simulink library "SimplusGT"  (R2022b)
settings: Solver=ode45  StartTime=0.0  StopTime=10.0  RelTol=1e-3
values from neighbouring files (symbols this model uses):
  ang_r = u(3)    [Class_GridFollowingVSI.m]    (also in Class_GridFollowingVSI_Disturb.m; Class_GridFollowingVSI_old.m)
  Cf = obj.Para(3)    [Class_GridFormingVSI.m]
  Lc = obj.Para(4)    [Class_GridFormingVSI.m]
  Lf = obj.Para(1)    [Class_GridFormingVSI.m]
  P_dc = u(4)    [Class_GridFollowingVSI.m]    (also in Class_GridFollowingVSI_Disturb.m; Class_GridFollowingVSI_old.m)
  Ts = []    [Class_Model_Advance.m]
  V = obj.PowerFlow(3)    [Class_GridFollowingVSI.m]    (also in Class_GridFollowingVSI_Disturb.m; Class_GridFollowingVSI_old.m; Class_GridFormingVSI.m; Class_InfiniteBus.m)
  x0 = []    [Class_Model_Advance.m]
undefined symbols (not defined in the file or in its folder): DiscIntNeverNeededParam, initial, m, OtherInputs, Sbase, t0, Tm_pu, Vbase, w_droop, w_i, w_pll, w_tau, w_v, Wbase, wc, wfil, Ybase, Zbase
libraries: spsVoltageMeasurementLib x107, spsCurrentMeasurementLib x92, spsControlledCurrentSourceLib x57, spsThreePhaseSeriesRLCBranchLib x29, spsControlledVoltageSourceLib x19, spsSeriesRLCBranchLib x15, SimplexPS_2015a x6, spsThreePhaseParallelRLCBranchLib x3, spsThreePhaseBreakerLib x2, $bdroot x1
(part 4 of 8)

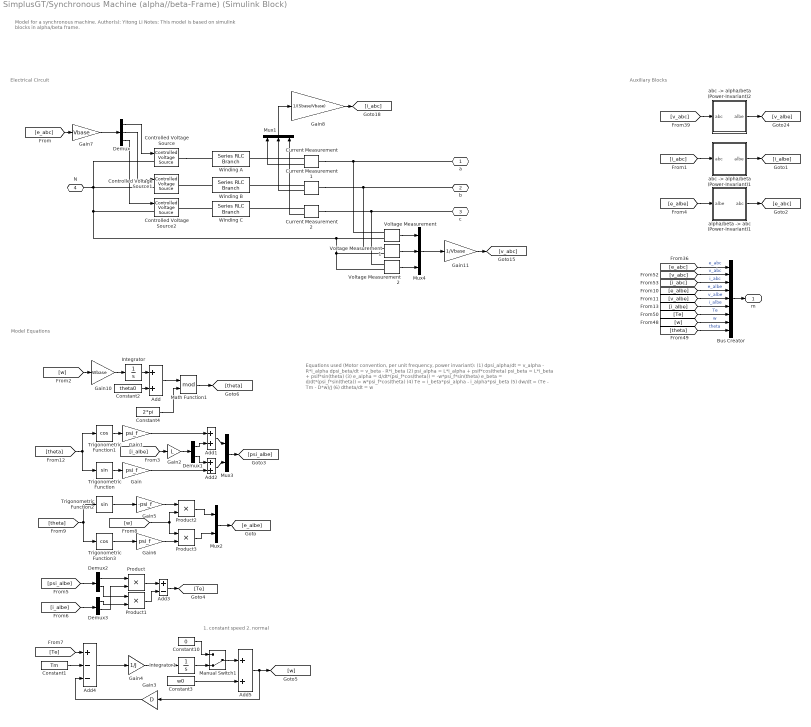
== system SimplusGT/Synchronous Machine (alpha//beta-Frame) (Simulink Block) ==
  note: 1. constant speed
      | 2. normal
  note: Auxiliary Blocks
  note: Model Equations
  note: Electrical Circuit
  note: Equations used
      | (Motor convention, per unit frequency, power invariant):
      |
      | (1) dpsi_alpha/dt = v_alpha - R*i_alpha
      | dpsi_beta/dt = v_beta - R*i_beta
      |
      | (2) psi_alpha = L*i_alpha + psif*cos(theta)
      | psi_beta = L*i_beta + psif*sin(theta)
      |
      | (3) e_alpha = d/dt*(psi_f*cos(theta)) = -w*psi_f*sin(theta)
      | e_beta = d/dt*(psi_f*sin(theta)) = w*psi_f*cos(theta)
      |
      | (4) Te = i_beta*psi_alpha - i_alpha*psi_beta
      | (5) dw/dt = (Te - Tm - D*w)/J
      | (6) dtheta/dt = w
  note: Model for a synchronous machine.
      |
      | Author(s): Yitong Li
      |
      | Notes:
      |
      | This model is based on simulink blocks in alpha/beta frame.
  Add{,1..2,5} (4 alike) : Sum
  Add3 : Sum  Inputs=+-
  Add4 : Sum  Inputs=+--
  Bus Creator : BusCreator  Inputs=9
  Constant1 : Constant  Value=Tm
  Constant10 : Constant  Value=0
  Constant2 : Constant  Value=theta0
  Constant3 : Constant  Value=w0
  Constant4 : Constant  Value=2*pi
  Controlled Voltage Source : spsControlledVoltageSourceLib/Controlled Voltage Source  Initialize=on  Source_Type=AC  Amplitude=0  Phase=0  Frequency=0  Measurements=None
  Controlled Voltage Source1 : spsControlledVoltageSourceLib/Controlled Voltage Source  Initialize=on  Source_Type=AC  Amplitude=0  Phase=0  Frequency=0  Measurements=None
  Controlled Voltage Source2 : spsControlledVoltageSourceLib/Controlled Voltage Source  Initialize=on  Source_Type=AC  Amplitude=0  Phase=0  Frequency=0  Measurements=None
  Current Measurement : spsCurrentMeasurementLib/Current Measurement  PhasorSimulation=off  OutputType=Complex  PSBequivalent=0
  Current Measurement1 : spsCurrentMeasurementLib/Current Measurement  PhasorSimulation=off  OutputType=Complex  PSBequivalent=0
  Current Measurement2 : spsCurrentMeasurementLib/Current Measurement  PhasorSimulation=off  OutputType=Complex  PSBequivalent=0
  Demux : Demux  Outputs=3
  Demux1 : Demux  Outputs=2
  Demux2 : Demux  Outputs=2
  Demux3 : Demux  Outputs=2
  Gain : Gain  Gain=psi_f
  Gain1 : Gain  Gain=psi_f
  Gain10 : Gain  Gain=Wbase
  Gain11 : Gain  Gain=1/Vbase
  Gain2 : Gain  Gain=L
  Gain3 : Gain  Gain=D
  Gain4 : Gain  Gain=1/J
  Gain5 : Gain  Gain=-psi_f
  Gain6 : Gain  Gain=psi_f
  Gain7 : Gain  Gain=Vbase
  Gain8 : Gain  Gain=1/(Sbase/Vbase)
  Integrator : Integrator
  Integrator1 : Integrator
  Manual Switch1 : ManualSwitch  CurrentSetting=0
  Math Function1 : Math  Operator=mod  SignedPower=on
  Mux1 : Mux  Inputs=3
  Mux2 : Mux  Inputs=2
  Mux3 : Mux  Inputs=2
  Mux4 : Mux  Inputs=3
  Product{,1..3} (4 alike) : Product
  Trigonometric Function : Trigonometry
  Trigonometric Function1 : Trigonometry  Operator=cos
  Trigonometric Function2 : Trigonometry
  Trigonometric Function3 : Trigonometry  Operator=cos
  Voltage Measurement : spsVoltageMeasurementLib/Voltage Measurement  PhasorSimulation=off  OutputType=Complex  PSBequivalent=0
  Voltage Measurement1 : spsVoltageMeasurementLib/Voltage Measurement  PhasorSimulation=off  OutputType=Complex  PSBequivalent=0
  Voltage Measurement2 : spsVoltageMeasurementLib/Voltage Measurement  PhasorSimulation=off  OutputType=Complex  PSBequivalent=0
  Winding A : spsSeriesRLCBranchLib/Series RLC Branch  LConnTagsString=__new0  RConnTagsString=__new0  BranchType=RL  Resistance=R*(Vbase^2)/Sbase  Inductance=L*(Vbase^2)/Sbase/Wbase  SetiL0=off  InitialCurrent=ia0  Capacitance=1e-6  Setx0=off  InitialVoltage=0  Measurements=None
  Winding B : spsSeriesRLCBranchLib/Series RLC Branch  LConnTagsString=__new0  RConnTagsString=__new0  BranchType=RL  Resistance=R*(Vbase^2)/Sbase  Inductance=L*(Vbase^2)/Sbase/Wbase  SetiL0=off  InitialCurrent=ia0  Capacitance=1e-6  Setx0=off  InitialVoltage=0  Measurements=None
  Winding C : spsSeriesRLCBranchLib/Series RLC Branch  LConnTagsString=__new0  RConnTagsString=__new0  BranchType=RL  Resistance=R*(Vbase^2)/Sbase  Inductance=L*(Vbase^2)/Sbase/Wbase  SetiL0=off  InitialCurrent=ia0  Capacitance=1e-6  Setx0=off  InitialVoltage=0  Measurements=None
  "abc -> alpha/beta (Power-Invariant)1" : Subsystem  AncestorBlock=|
      | SimplusGT/abc -> alpha//beta
      | (Power-Invariant)
      settings: LibrarySourceBlock=|
      | SimplusGT/abc -> alpha//beta
      | (Power-Invariant)
  "abc -> alpha/beta (Power-Invariant)2" : Subsystem  AncestorBlock=|
      | SimplusGT/abc -> alpha//beta
      | (Power-Invariant)
      settings: LibrarySourceBlock=|
      | SimplusGT/abc -> alpha//beta
      | (Power-Invariant)
  "alpha/beta -> abc (Power-Invariant)1" : Subsystem  AncestorBlock=|
      | SimplusGT/alpha//beta -> abc
      | (Power-Invariant)
      settings: LibrarySourceBlock=|
      | SimplusGT/alpha//beta -> abc
      | (Power-Invariant)
  a : PMIOPort  Side=Left
  b : PMIOPort  Port=2  Side=Left
  c : PMIOPort  Port=3  Side=Left
  N : PMIOPort  Port=4  Side=Left
  m : Outport
  wires:
  Current Measurement/1 -> Mux1/1
  Current Measurement1/1 -> Mux1/2
  Current Measurement2/1 -> Mux1/3
  Mux1/1 -> Gain8/1
  [e_abc] -> Gain7/1
  Demux/1 -> Controlled Voltage Source/1
  Demux/2 -> Controlled Voltage Source1/1
  Demux/3 -> Controlled Voltage Source2/1
  [i_abc] -> "abc -> alpha/beta (Power-Invariant)1"/1(abc)
  "abc -> alpha/beta (Power-Invariant)1"/1(albe) -> [i_albe]
  [w] -> Gain10/1
  Integrator/1 -> Add/1
  Constant2/1 -> Add/2
  Trigonometric Function1/1 -> Gain1/1
  Trigonometric Function/1 -> Gain/1
  [i_albe] -> Gain2/1
  Demux1/1 -> Add1/2
  Demux1/2 -> Add2/1
  Gain2/1 -> Demux1/1
  Gain1/1 -> Add1/1
  Gain/1 -> Add2/2
  Product2/1 -> Mux2/1
  Product3/1 -> Mux2/2
  Mux2/1 -> [e_albe]
  [e_albe] -> "alpha/beta -> abc (Power-Invariant)1"/1(albe)
  "alpha/beta -> abc (Power-Invariant)1"/1(abc) -> [e_abc]
  Add1/1 -> Mux3/1
  Add2/1 -> Mux3/2
  Mux3/1 -> [psi_albe]
  [psi_albe] -> Demux2/1
  [i_albe] -> Demux3/1
  Demux2/1 -> Product/1
  Demux3/2 -> Product/2
  Demux3/1 -> Product1/2
  Demux2/2 -> Product1/1
  Product/1 -> Add3/1
  Product1/1 -> Add3/2
  Add3/1 -> [Te]
  [Te] -> Add4/1
  Constant1/1 -> Add4/2
  Add4/1 -> Gain4/1
  Gain3/1 -> Add4/3
  Constant3/1 -> Add5/2
  Add5/1 -> Gain3/1, [w]
  [theta] -> Trigonometric Function3/1, Trigonometric Function2/1
  Trigonometric Function2/1 -> Gain5/1
  Trigonometric Function3/1 -> Gain6/1
  Gain5/1 -> Product2/1
  Gain6/1 -> Product3/2
  Gain8/1 -> [i_abc]
  Gain4/1 -> Integrator1/1
  Gain10/1 -> Integrator/1
  Voltage Measurement/1 -> Mux4/1
  Voltage Measurement1/1 -> Mux4/2
  Voltage Measurement2/1 -> Mux4/3
  Mux4/1 -> Gain11/1
  Gain11/1 -> [v_abc]
  Gain7/1 -> Demux/1
  Add/1 -> Math Function1/1
  Constant4/1 -> Math Function1/2
  Math Function1/1 -> [theta]
  [v_abc] -> "abc -> alpha/beta (Power-Invariant)2"/1(abc)
  "abc -> alpha/beta (Power-Invariant)2"/1(albe) -> [v_albe]
  [w] -> Product3/1, Product2/2
  [theta] -> Trigonometric Function/1, Trigonometric Function1/1
  Integrator1/1 -> Manual Switch1/2
  Manual Switch1/1 -> Add5/1
  Constant10/1 -> Manual Switch1/1
  [e_abc] -> Bus Creator/1  "e_abc"
  [v_abc] -> Bus Creator/2  "v_abc"
  [i_abc] -> Bus Creator/3  "i_abc"
  [e_albe] -> Bus Creator/4  "e_albe"
  [v_albe] -> Bus Creator/5  "v_albe"
  [i_albe] -> Bus Creator/6  "i_albe"
  [Te] -> Bus Creator/7  "Te"
  [w] -> Bus Creator/8  "w"
  [theta] -> Bus Creator/9  "theta"
  Bus Creator/1 -> m/1
  connections:
  Current Measurement/RConn1 -- Winding A/RConn1
  Controlled Voltage Source/RConn1 -- Winding A/LConn1
  Current Measurement2/RConn1 -- Winding C/RConn1
  Current Measurement/LConn1 -- Voltage Measurement/LConn1 -- a/RConn1
  Current Measurement1/LConn1 -- Voltage Measurement1/LConn1 -- b/RConn1
  Current Measurement1/RConn1 -- Winding B/RConn1
  Winding B/LConn1 -- Controlled Voltage Source1/RConn1
  Controlled Voltage Source/LConn1 -- Voltage Measurement2/LConn2 -- Voltage Measurement1/LConn2 -- Voltage Measurement/LConn2 -- Controlled Voltage Source2/LConn1 -- N/RConn1 -- Controlled Voltage Source1/LConn1
  Winding C/LConn1 -- Controlled Voltage Source2/RConn1
  Current Measurement2/LConn1 -- Voltage Measurement2/LConn1 -- c/RConn1

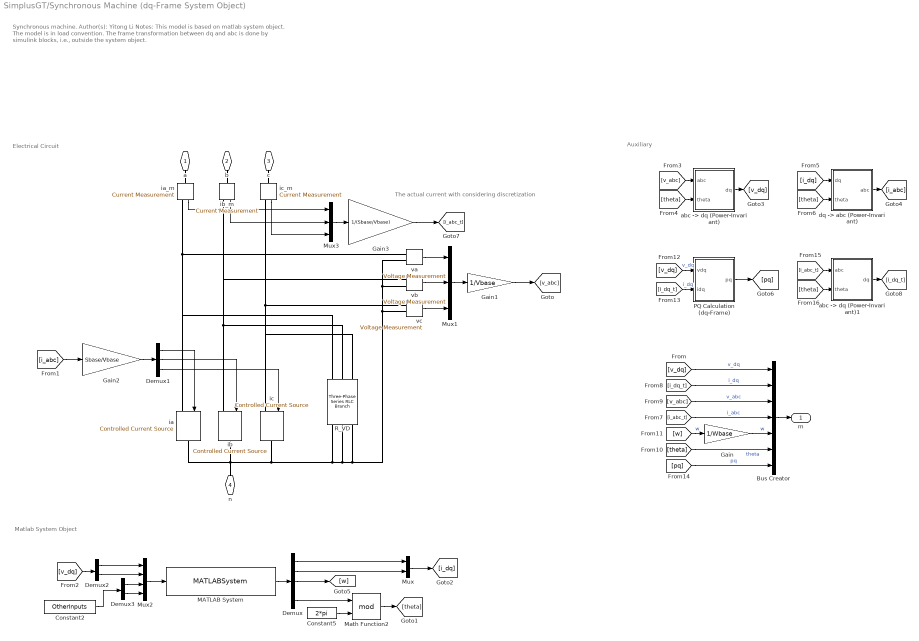
== system SimplusGT/Synchronous Machine (dq-Frame System Object) ==
  note: The actual current with considering discretization
  note: Synchronous machine.
      |
      | Author(s): Yitong Li
      |
      | Notes:
      |
      | This model is based on matlab system object.
      |
      | The model is in load convention.
      |
      | The frame transformation between dq and abc is done by simulink blocks, i.e., outside the system object.
  note: Matlab System Object
  note: Auxiliary
  note: Electrical Circuit
  Bus Creator : BusCreator  Inputs=7
  Constant2 : Constant  Value=OtherInputs
  Constant5 : Constant  Value=2*pi
  Demux : Demux  Outputs=5
  Demux1 : Demux  Outputs=3
  Demux2 : Demux  Outputs=2
  Demux3 : Demux  Outputs=2
  Gain : Gain  Gain=1/Wbase
  Gain1 : Gain  Gain=1/Vbase
  Gain2 : Gain  Gain=Sbase/Vbase
  Gain3 : Gain  Gain=1/(Sbase/Vbase)
  MATLAB System : MATLABSystem  System=SimplusGT.Class.SynchronousMachine  Ts=Ts  Para=ApparatusPara  ApparatusType=ApparatusType  PowerFlow=PowerFlow  x0=x0  DiscreMethod=DiscreMethod  LinearizationTimes=LinearizationTimes  DirectFeedthrough=DirectFeedthrough  VirtualResistor=DiscreDampingFlag  EquiInitial=true  ElecPortIOs=[ 1, 2 ]  SimulateUsing=Code generation
      mask Type: SimplusGT.Class.SynchronousMachine
      mask Display:
      | disp('SynchronousMachine');
      | port_label('input',1,'u');
      | port_label('output',1,'y');
  Math Function2 : Math  Operator=mod  SignedPower=on
  Mux : Mux  Inputs=2
  Mux1 : Mux  Inputs=3
  Mux2 : Mux
  Mux3 : Mux  Inputs=3
  PQ Calculation (dq-Frame) : Subsystem  AncestorBlock=|
      | SimplusGT/PQ Calculation
      | (dq-Frame)
      settings: LibrarySourceBlock=|
      | SimplusGT/PQ Calculation
      | (dq-Frame)
  R_VD : spsThreePhaseSeriesRLCBranchLib/Three-Phase Series RLC Branch  LConnTagsString=A|B|C  RConnTagsString=A|B|C  BranchType=R  Resistance=DiscreDampingValue*Vbase^2/Sbase  Inductance=1e-3  Capacitance=1e-6  Measurements=None
  "abc -> dq (Power-Invariant)" : Subsystem  AncestorBlock=|
      | SimplusGT/abc -> dq
      | (Power-Invariant)
      settings: LibrarySourceBlock=|
      | SimplusGT/abc -> dq
      | (Power-Invariant)
  "abc -> dq (Power-Invariant)1" : Subsystem  AncestorBlock=|
      | SimplusGT/abc -> dq
      | (Power-Invariant)
      settings: LibrarySourceBlock=|
      | SimplusGT/abc -> dq
      | (Power-Invariant)
  "dq -> abc (Power-Invariant)" : Subsystem  AncestorBlock=|
      | SimplusGT/dq -> abc
      | (Power-Invariant)
      settings: LibrarySourceBlock=|
      | SimplusGT/dq -> abc
      | (Power-Invariant)
  ia : spsControlledCurrentSourceLib/Controlled Current Source  Initialize=on  Source_Type=AC  Amplitude=0  Phase=0  Frequency=0  Measurements=None
  ia_m : spsCurrentMeasurementLib/Current Measurement  PhasorSimulation=off  OutputType=Complex  PSBequivalent=0
  ib : spsControlledCurrentSourceLib/Controlled Current Source  Initialize=on  Source_Type=AC  Amplitude=0  Phase=0  Frequency=0  Measurements=None
  ib_m : spsCurrentMeasurementLib/Current Measurement  PhasorSimulation=off  OutputType=Complex  PSBequivalent=0
  ic : spsControlledCurrentSourceLib/Controlled Current Source  Initialize=on  Source_Type=AC  Amplitude=0  Phase=0  Frequency=0  Measurements=None
  ic_m : spsCurrentMeasurementLib/Current Measurement  PhasorSimulation=off  OutputType=Complex  PSBequivalent=0
  va : spsVoltageMeasurementLib/Voltage Measurement  PhasorSimulation=off  OutputType=Complex  PSBequivalent=0
  vb : spsVoltageMeasurementLib/Voltage Measurement  PhasorSimulation=off  OutputType=Complex  PSBequivalent=0
  vc : spsVoltageMeasurementLib/Voltage Measurement  PhasorSimulation=off  OutputType=Complex  PSBequivalent=0
  a : PMIOPort  Side=Left
  b : PMIOPort  Port=2  Side=Left
  c : PMIOPort  Port=3  Side=Left
  n : PMIOPort  Port=4  Side=Left
  m : Outport
  wires:
  Demux/2 -> Mux/2
  Demux/1 -> Mux/1
  Mux/1 -> [i_dq]
  Demux/3 -> [w]
  Demux1/1 -> ia/1
  Demux1/2 -> ib/1
  va/1 -> Mux1/1
  vb/1 -> Mux1/2
  [v_dq] -> Demux2/1
  Demux2/1 -> Mux2/1
  Demux2/2 -> Mux2/2
  [v_abc] -> "abc -> dq (Power-Invariant)"/1(abc)
  [theta] -> "abc -> dq (Power-Invariant)"/2(theta)
  "abc -> dq (Power-Invariant)"/1(dq) -> [v_dq]
  [i_dq] -> "dq -> abc (Power-Invariant)"/1(dq)
  [theta] -> "dq -> abc (Power-Invariant)"/2(theta)
  "dq -> abc (Power-Invariant)"/1(abc) -> [i_abc]
  Mux2/1 -> MATLAB System/1
  MATLAB System/1 -> Demux/1
  vc/1 -> Mux1/3
  Demux1/3 -> ic/1
  Demux/5 -> Math Function2/1
  Constant5/1 -> Math Function2/2
  Math Function2/1 -> [theta]
  [v_dq] -> Bus Creator/1  "v_dq"
  [i_dq_t] -> Bus Creator/2  "i_dq"
  [v_abc] -> Bus Creator/3  "v_abc"
  [i_abc_t] -> Bus Creator/4  "i_abc"
  [w] -> Gain/1  "w"
  [theta] -> Bus Creator/6  "theta"
  Bus Creator/1 -> m/1
  Gain/1 -> Bus Creator/5  "w"
  Mux1/1 -> Gain1/1
  Constant2/1 -> Demux3/1
  Demux3/1 -> Mux2/3
  Demux3/2 -> Mux2/4
  [i_abc] -> Gain2/1
  [v_dq] -> PQ Calculation (dq-Frame)/1(vdq)  "v_dq"
  [i_dq_t] -> PQ Calculation (dq-Frame)/2(idq)  "i_dq"
  PQ Calculation (dq-Frame)/1(pq) -> [pq]
  [pq] -> Bus Creator/7  "pq"
  Gain1/1 -> [v_abc]
  Gain2/1 -> Demux1/1
  ia_m/1 -> Mux3/1
  ib_m/1 -> Mux3/2
  ic_m/1 -> Mux3/3
  Mux3/1 -> Gain3/1
  Gain3/1 -> [i_abc_t]
  [i_abc_t] -> "abc -> dq (Power-Invariant)1"/1(abc)
  [theta] -> "abc -> dq (Power-Invariant)1"/2(theta)
  "abc -> dq (Power-Invariant)1"/1(dq) -> [i_dq_t]
  connections:
  vb/LConn2 -- va/LConn2 -- vc/LConn2 -- R_VD/RConn3 -- R_VD/RConn2 -- R_VD/RConn1 -- ia/RConn1 -- ib/RConn1 -- n/RConn1 -- ic/RConn1
  R_VD/LConn2 -- vb/LConn1 -- ib_m/RConn1 -- ib/LConn1
  R_VD/LConn3 -- ic/LConn1 -- ic_m/RConn1 -- vc/LConn1
  va/LConn1 -- R_VD/LConn1 -- ia/LConn1 -- ia_m/RConn1
  ia_m/LConn1 -- a/RConn1
  ib_m/LConn1 -- b/RConn1
  ic_m/LConn1 -- c/RConn1

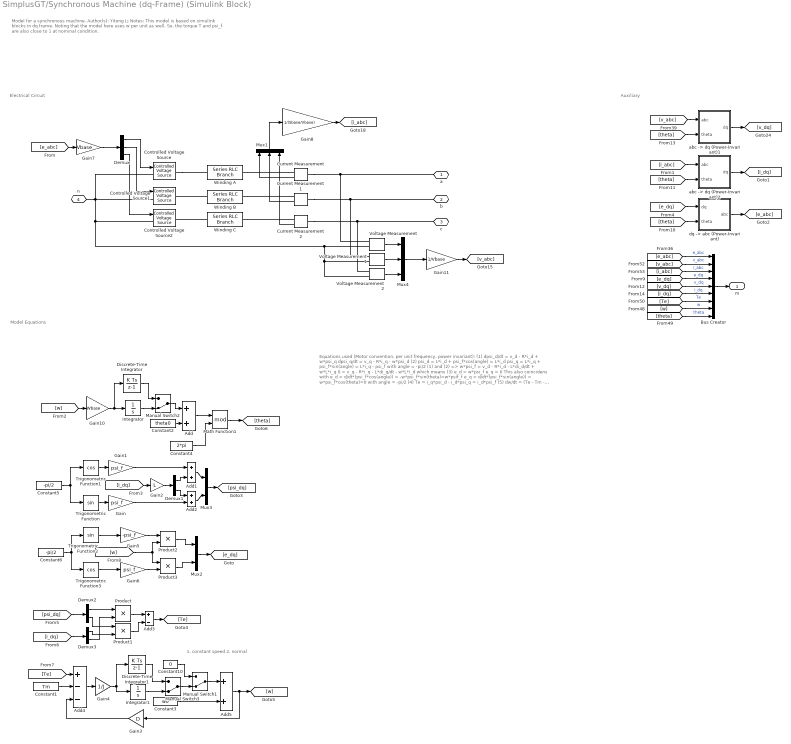
== system SimplusGT/Synchronous Machine (dq-Frame) (Simulink Block) ==
  note: 1. constant speed
      | 2. normal
  note: Auxiliary
  note: Model Equations
  note: Electrical Circuit
  note: Equations used
      | (Motor convention, per unit frequency, power invariant):
      |
      | (1) dpsi_d/dt = v_d - R*i_d + w*psi_q
      | dpsi_q/dt = v_q - R*i_q - w*psi_d
      |
      | (2) psi_d = L*i_d + psi_f*cos(angle) = L*i_d
      | psi_q = L*i_q + psi_f*sin(angle) = L*i_q - psi_f
      | with angle = -pi/2
      |
      | (1) and (2) =>
      |
      | w*psi_f = v_d - R*i_d - L*di_d/dt + w*L*i_q
      | 0 = v_q - R*i_q - L*di_q/dt - w*L*i_d
      |
      | which means
      |
      | (3) e_d = w*psi_f
      | e_q = 0
      |
      | This also coincidens with
      |
      | e_d = d/dt*(psi_f*cos(angle)) = -w*psi_f*sin(theta)=w*psif_f
      | e_q = d/dt*(psi_f*sin(angle)) = w*psi_f*cos(theta)=0
      | with angle = -pi/2
      |
      | (4) Te = i_q*psi_d - i_d*psi_q = i_d*psi_f
      | (5) dw/dt = (Te - Tm - D*w)/J
      | (6) dtheta/dt = w
  note: Model for a synchronous machine.
      |
      | Author(s): Yitong Li
      |
      | Notes:
      |
      | This model is based on simulink blocks in dq frame.
      |
      | Noting that the model here uses w per unit as well. So, the torque T and psi_f are also close to 1 at nominal condition.
  Add{,1..2,5} (4 alike) : Sum
  Add3 : Sum  Inputs=+-
  Add4 : Sum  Inputs=+--
  Bus Creator : BusCreator  Inputs=9
  Constant1 : Constant  Value=Tm
  Constant10 : Constant  Value=0
  Constant2 : Constant  Value=theta0
  Constant3 : Constant  Value=w0
  Constant4 : Constant  Value=2*pi
  Constant5 : Constant  Value=-pi/2
  Constant6 : Constant  Value=-pi/2
  Controlled Voltage Source : spsControlledVoltageSourceLib/Controlled Voltage Source  Initialize=on  Source_Type=AC  Amplitude=0  Phase=0  Frequency=0  Measurements=None
  Controlled Voltage Source1 : spsControlledVoltageSourceLib/Controlled Voltage Source  Initialize=on  Source_Type=AC  Amplitude=0  Phase=0  Frequency=0  Measurements=None
  Controlled Voltage Source2 : spsControlledVoltageSourceLib/Controlled Voltage Source  Initialize=on  Source_Type=AC  Amplitude=0  Phase=0  Frequency=0  Measurements=None
  Current Measurement : spsCurrentMeasurementLib/Current Measurement  PhasorSimulation=off  OutputType=Complex  PSBequivalent=0
  Current Measurement1 : spsCurrentMeasurementLib/Current Measurement  PhasorSimulation=off  OutputType=Complex  PSBequivalent=0
  Current Measurement2 : spsCurrentMeasurementLib/Current Measurement  PhasorSimulation=off  OutputType=Complex  PSBequivalent=0
  Demux : Demux  Outputs=3
  Demux1 : Demux  Outputs=2
  Demux2 : Demux  Outputs=2
  Demux3 : Demux  Outputs=2
  Discrete-Time Integrator : DiscreteIntegrator  SampleTime=-1  ICPrevOutput=DiscIntNeverNeededParam  ICPrevScaledInput=DiscIntNeverNeededParam
  Discrete-Time Integrator1 : DiscreteIntegrator  SampleTime=-1  ICPrevOutput=DiscIntNeverNeededParam  ICPrevScaledInput=DiscIntNeverNeededParam
  Gain : Gain  Gain=psi_f
  Gain1 : Gain  Gain=psi_f
  Gain10 : Gain  Gain=Wbase
  Gain11 : Gain  Gain=1/Vbase
  Gain2 : Gain  Gain=L
  Gain3 : Gain  Gain=D
  Gain4 : Gain  Gain=1/J
  Gain5 : Gain  Gain=-psi_f
  Gain6 : Gain  Gain=psi_f
  Gain7 : Gain  Gain=Vbase
  Gain8 : Gain  Gain=1/(Sbase/Vbase)
  Integrator : Integrator
  Integrator1 : Integrator
  Manual Switch1 : ManualSwitch  CurrentSetting=0
  Manual Switch2 : ManualSwitch  CurrentSetting=0
  Manual Switch3 : ManualSwitch  CurrentSetting=0
  Math Function1 : Math  Operator=mod  SignedPower=on
  Mux1 : Mux  Inputs=3
  Mux2 : Mux  Inputs=2
  Mux3 : Mux  Inputs=2
  Mux4 : Mux  Inputs=3
  Product{,1..3} (4 alike) : Product
  Trigonometric Function : Trigonometry
  Trigonometric Function1 : Trigonometry  Operator=cos
  Trigonometric Function2 : Trigonometry
  Trigonometric Function3 : Trigonometry  Operator=cos
  Voltage Measurement : spsVoltageMeasurementLib/Voltage Measurement  PhasorSimulation=off  OutputType=Complex  PSBequivalent=0
  Voltage Measurement1 : spsVoltageMeasurementLib/Voltage Measurement  PhasorSimulation=off  OutputType=Complex  PSBequivalent=0
  Voltage Measurement2 : spsVoltageMeasurementLib/Voltage Measurement  PhasorSimulation=off  OutputType=Complex  PSBequivalent=0
  Winding A : spsSeriesRLCBranchLib/Series RLC Branch  LConnTagsString=__new0  RConnTagsString=__new0  BranchType=RL  Resistance=R*(Vbase^2)/Sbase  Inductance=L*(Vbase^2)/Sbase/Wbase  SetiL0=off  InitialCurrent=ia0  Capacitance=1e-6  Setx0=off  InitialVoltage=0  Measurements=None
  Winding B : spsSeriesRLCBranchLib/Series RLC Branch  LConnTagsString=__new0  RConnTagsString=__new0  BranchType=RL  Resistance=R*(Vbase^2)/Sbase  Inductance=L*(Vbase^2)/Sbase/Wbase  SetiL0=off  InitialCurrent=ia0  Capacitance=1e-6  Setx0=off  InitialVoltage=0  Measurements=None
  Winding C : spsSeriesRLCBranchLib/Series RLC Branch  LConnTagsString=__new0  RConnTagsString=__new0  BranchType=RL  Resistance=R*(Vbase^2)/Sbase  Inductance=L*(Vbase^2)/Sbase/Wbase  SetiL0=off  InitialCurrent=ia0  Capacitance=1e-6  Setx0=off  InitialVoltage=0  Measurements=None
  "abc -> dq (Power-Invariant)1" : Subsystem  AncestorBlock=|
      | SimplusGT/Synchronous Machine
      | (dq-Frame System Object)/abc -> dq
      | (Power-Invariant)
      settings: LibrarySourceBlock=|
      | SimplusGT/Synchronous Machine
      | (dq-Frame System Object)/abc -> dq
      | (Power-Invariant)
  "abc -> dq (Power-Invariant)2" : Subsystem  AncestorBlock=|
      | SimplusGT/Synchronous Machine
      | (dq-Frame)
      | (Simulink Block)/abc -> dq
      | (Power-Invariant)1
      settings: LibrarySourceBlock=|
      | SimplusGT/Synchronous Machine
      | (dq-Frame)
      | (Simulink Block)/abc -> dq
      | (Power-Invariant)1
  "dq -> abc (Power-Invariant)" : Subsystem  AncestorBlock=|
      | SimplusGT/dq -> abc
      | (Power-Invariant)
      settings: LibrarySourceBlock=|
      | SimplusGT/dq -> abc
      | (Power-Invariant)
  a : PMIOPort  Side=Left
  b : PMIOPort  Port=2  Side=Left
  c : PMIOPort  Port=3  Side=Left
  n : PMIOPort  Port=4  Side=Left
  m : Outport
  wires:
  Current Measurement/1 -> Mux1/1
  Current Measurement1/1 -> Mux1/2
  Current Measurement2/1 -> Mux1/3
  Mux1/1 -> Gain8/1
  [e_abc] -> Gain7/1
  Demux/1 -> Controlled Voltage Source/1
  Demux/2 -> Controlled Voltage Source1/1
  Demux/3 -> Controlled Voltage Source2/1
  [i_abc] -> "abc -> dq (Power-Invariant)2"/1(abc)
  "abc -> dq (Power-Invariant)2"/1(dq) -> [i_dq]
  [w] -> Gain10/1
  Constant2/1 -> Add/2
  Trigonometric Function1/1 -> Gain1/1
  Trigonometric Function/1 -> Gain/1
  [i_dq] -> Gain2/1
  Demux1/1 -> Add1/2
  Demux1/2 -> Add2/1
  Gain2/1 -> Demux1/1
  Gain1/1 -> Add1/1
  Gain/1 -> Add2/2
  Product2/1 -> Mux2/1
  Product3/1 -> Mux2/2
  Mux2/1 -> [e_dq]
  [e_dq] -> "dq -> abc (Power-Invariant)"/1(dq)
  Add1/1 -> Mux3/1
  Add2/1 -> Mux3/2
  Mux3/1 -> [psi_dq]
  [psi_dq] -> Demux2/1
  [i_dq] -> Demux3/1
  Demux2/1 -> Product/1
  Demux3/2 -> Product/2
  Demux3/1 -> Product1/2
  Demux2/2 -> Product1/1
  Product/1 -> Add3/1
  Product1/1 -> Add3/2
  Add3/1 -> [Te]
  [Te] -> Add4/1
  Constant1/1 -> Add4/2
  Add4/1 -> Gain4/1
  Gain3/1 -> Add4/3
  Constant3/1 -> Add5/2
  Add5/1 -> Gain3/1, [w]
  Constant6/1 -> Trigonometric Function3/1, Trigonometric Function2/1
  Trigonometric Function2/1 -> Gain5/1
  Trigonometric Function3/1 -> Gain6/1
  Gain5/1 -> Product2/1
  Gain6/1 -> Product3/2
  Gain8/1 -> [i_abc]
  Gain4/1 -> Integrator1/1, Discrete-Time Integrator1/1
  Voltage Measurement/1 -> Mux4/1
  Voltage Measurement1/1 -> Mux4/2
  Voltage Measurement2/1 -> Mux4/3
  Mux4/1 -> Gain11/1
  Gain11/1 -> [v_abc]
  Gain7/1 -> Demux/1
  Add/1 -> Math Function1/1
  Constant4/1 -> Math Function1/2
  Math Function1/1 -> [theta]
  [v_abc] -> "abc -> dq (Power-Invariant)1"/1(abc)
  "abc -> dq (Power-Invariant)1"/1(dq) -> [v_dq]
  [w] -> Product3/1, Product2/2
  Constant5/1 -> Trigonometric Function/1, Trigonometric Function1/1
  Manual Switch1/1 -> Add5/1
  Constant10/1 -> Manual Switch1/1
  [theta] -> "dq -> abc (Power-Invariant)"/2(theta)
  [theta] -> "abc -> dq (Power-Invariant)2"/2(theta)
  [theta] -> "abc -> dq (Power-Invariant)1"/2(theta)
  [theta] -> Bus Creator/9  "theta"
  [e_dq] -> Bus Creator/4  "e_dq"
  [Te] -> Bus Creator/7  "Te"
  [i_abc] -> Bus Creator/3  "i_abc"
  [v_abc] -> Bus Creator/2  "v_abc"
  [v_dq] -> Bus Creator/5  "v_dq"
  [i_dq] -> Bus Creator/6  "i_dq"
  [e_abc] -> Bus Creator/1  "e_abc"
  [w] -> Bus Creator/8  "w"
  "dq -> abc (Power-Invariant)"/1(abc) -> [e_abc]
  Bus Creator/1 -> m/1
  Gain10/1 -> Discrete-Time Integrator/1, Integrator/1
  Integrator/1 -> Manual Switch2/2
  Manual Switch2/1 -> Add/1
  Discrete-Time Integrator/1 -> Manual Switch2/1
  Manual Switch3/1 -> Manual Switch1/2
  Integrator1/1 -> Manual Switch3/2
  Discrete-Time Integrator1/1 -> Manual Switch3/1
  connections:
  Current Measurement/RConn1 -- Winding A/RConn1
  Controlled Voltage Source/RConn1 -- Winding A/LConn1
  Current Measurement2/RConn1 -- Winding C/RConn1
  Current Measurement/LConn1 -- Voltage Measurement/LConn1 -- a/RConn1
  Current Measurement1/LConn1 -- Voltage Measurement1/LConn1 -- b/RConn1
  Current Measurement1/RConn1 -- Winding B/RConn1
  Winding B/LConn1 -- Controlled Voltage Source1/RConn1
  Controlled Voltage Source/LConn1 -- Voltage Measurement2/LConn2 -- Voltage Measurement1/LConn2 -- Voltage Measurement/LConn2 -- Controlled Voltage Source2/LConn1 -- n/RConn1 -- Controlled Voltage Source1/LConn1
  Winding C/LConn1 -- Controlled Voltage Source2/RConn1
  Current Measurement2/LConn1 -- Voltage Measurement2/LConn1 -- c/RConn1

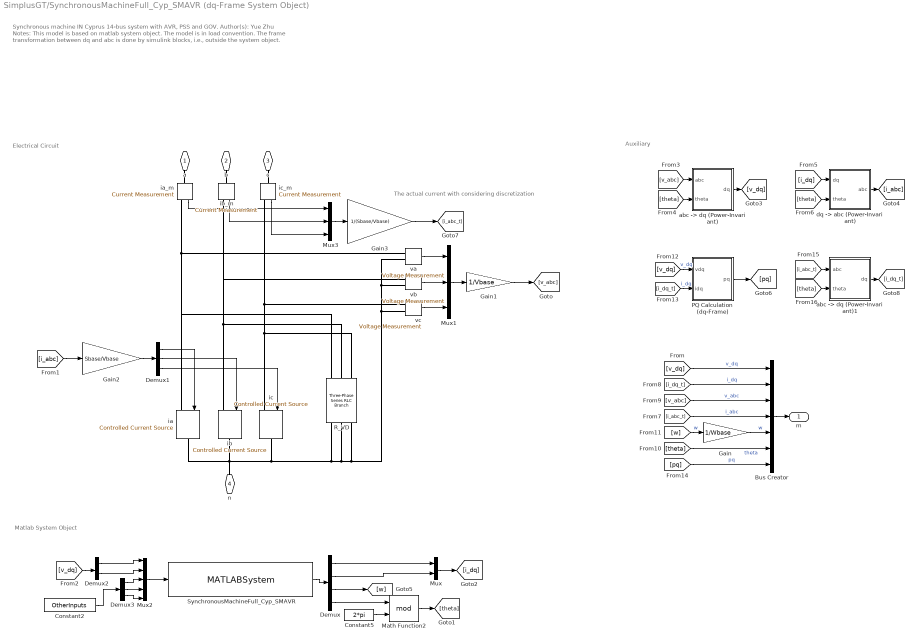
== system SimplusGT/SynchronousMachineFull_Cyp_SMAVR (dq-Frame System Object) ==
  note: The actual current with considering discretization
  note: Synchronous machine IN Cyprus 14-bus system with AVR, PSS and GOV.
      |
      | Author(s): Yue Zhu
      |
      | Notes:
      |
      | This model is based on matlab system object.
      |
      | The model is in load convention.
      |
      | The frame transformation between dq and abc is done by simulink blocks, i.e., outside the system object.
  note: Matlab System Object
  note: Auxiliary
  note: Electrical Circuit
  Bus Creator : BusCreator  Inputs=7
  Constant2 : Constant  Value=OtherInputs
  Constant5 : Constant  Value=2*pi
  Demux : Demux
  Demux1 : Demux  Outputs=3
  Demux2 : Demux  Outputs=2
  Demux3 : Demux  Outputs=3
  Gain : Gain  Gain=1/Wbase
  Gain1 : Gain  Gain=1/Vbase
  Gain2 : Gain  Gain=Sbase/Vbase
  Gain3 : Gain  Gain=1/(Sbase/Vbase)
  Math Function2 : Math  Operator=mod  SignedPower=on
  Mux : Mux  Inputs=2
  Mux1 : Mux  Inputs=3
  Mux2 : Mux  Inputs=5
  Mux3 : Mux  Inputs=3
  PQ Calculation (dq-Frame) : Subsystem  AncestorBlock=|
      | SimplusGT/PQ Calculation
      | (dq-Frame)
      settings: LibrarySourceBlock=|
      | SimplusGT/PQ Calculation
      | (dq-Frame)
  R_VD : spsThreePhaseSeriesRLCBranchLib/Three-Phase Series RLC Branch  LConnTagsString=A|B|C  RConnTagsString=A|B|C  BranchType=R  Resistance=DiscreDampingValue*Vbase^2/Sbase  Inductance=1e-3  Capacitance=1e-6  Measurements=None
  SynchronousMachineFull_Cyp_SMAVR : MATLABSystem  System=SimplusGT.Class.SynchronousMachineFull_Cyp_SMAVR  Ts=Ts  Para=ApparatusPara  ApparatusType=ApparatusType  PowerFlow=PowerFlow  x0=x0  DiscreMethod=DiscreMethod  LinearizationTimes=LinearizationTimes  DirectFeedthrough=DirectFeedthrough  VirtualResistor=DiscreDampingFlag  EquiInitial=true  ElecPortIOs=[ 1, 2 ]  SimulateUsing=Code generation
      mask Type: SimplusGT.Class.SynchronousMachineFull_Cyp_SMAVR
      mask Display:
      | disp('SynchronousMachineFull_Cyp_SMAVR');
      | port_label('input',1,'u');
      | port_label('output',1,'y');
  "abc -> dq (Power-Invariant)" : Subsystem  AncestorBlock=|
      | SimplusGT/abc -> dq
      | (Power-Invariant)
      settings: LibrarySourceBlock=|
      | SimplusGT/abc -> dq
      | (Power-Invariant)
  "abc -> dq (Power-Invariant)1" : Subsystem  AncestorBlock=|
      | SimplusGT/abc -> dq
      | (Power-Invariant)
      settings: LibrarySourceBlock=|
      | SimplusGT/abc -> dq
      | (Power-Invariant)
  "dq -> abc (Power-Invariant)" : Subsystem  AncestorBlock=|
      | SimplusGT/dq -> abc
      | (Power-Invariant)
      settings: LibrarySourceBlock=|
      | SimplusGT/dq -> abc
      | (Power-Invariant)
  ia : spsControlledCurrentSourceLib/Controlled Current Source  Initialize=on  Source_Type=AC  Amplitude=0  Phase=0  Frequency=0  Measurements=None
  ia_m : spsCurrentMeasurementLib/Current Measurement  PhasorSimulation=off  OutputType=Complex  PSBequivalent=0
  ib : spsControlledCurrentSourceLib/Controlled Current Source  Initialize=on  Source_Type=AC  Amplitude=0  Phase=0  Frequency=0  Measurements=None
  ib_m : spsCurrentMeasurementLib/Current Measurement  PhasorSimulation=off  OutputType=Complex  PSBequivalent=0
  ic : spsControlledCurrentSourceLib/Controlled Current Source  Initialize=on  Source_Type=AC  Amplitude=0  Phase=0  Frequency=0  Measurements=None
  ic_m : spsCurrentMeasurementLib/Current Measurement  PhasorSimulation=off  OutputType=Complex  PSBequivalent=0
  va : spsVoltageMeasurementLib/Voltage Measurement  PhasorSimulation=off  OutputType=Complex  PSBequivalent=0
  vb : spsVoltageMeasurementLib/Voltage Measurement  PhasorSimulation=off  OutputType=Complex  PSBequivalent=0
  vc : spsVoltageMeasurementLib/Voltage Measurement  PhasorSimulation=off  OutputType=Complex  PSBequivalent=0
  a : PMIOPort  Side=Left
  b : PMIOPort  Port=2  Side=Left
  c : PMIOPort  Port=3  Side=Left
  n : PMIOPort  Port=4  Side=Left
  m : Outport
  wires:
  Demux/2 -> Mux/2
  Demux/1 -> Mux/1
  Mux/1 -> [i_dq]
  Demux/3 -> [w]
  Demux1/1 -> ia/1
  Demux1/2 -> ib/1
  va/1 -> Mux1/1
  vb/1 -> Mux1/2
  [v_dq] -> Demux2/1
  Demux2/1 -> Mux2/1
  Demux2/2 -> Mux2/2
  [v_abc] -> "abc -> dq (Power-Invariant)"/1(abc)
  [theta] -> "abc -> dq (Power-Invariant)"/2(theta)
  "abc -> dq (Power-Invariant)"/1(dq) -> [v_dq]
  [i_dq] -> "dq -> abc (Power-Invariant)"/1(dq)
  [theta] -> "dq -> abc (Power-Invariant)"/2(theta)
  "dq -> abc (Power-Invariant)"/1(abc) -> [i_abc]
  Mux2/1 -> SynchronousMachineFull_Cyp_SMAVR/1
  SynchronousMachineFull_Cyp_SMAVR/1 -> Demux/1
  vc/1 -> Mux1/3
  Demux1/3 -> ic/1
  Demux/4 -> Math Function2/1
  Constant5/1 -> Math Function2/2
  Math Function2/1 -> [theta]
  [v_dq] -> Bus Creator/1  "v_dq"
  [i_dq_t] -> Bus Creator/2  "i_dq"
  [v_abc] -> Bus Creator/3  "v_abc"
  [i_abc_t] -> Bus Creator/4  "i_abc"
  [w] -> Gain/1  "w"
  [theta] -> Bus Creator/6  "theta"
  Bus Creator/1 -> m/1
  Gain/1 -> Bus Creator/5  "w"
  Mux1/1 -> Gain1/1
  Constant2/1 -> Demux3/1
  Demux3/1 -> Mux2/3
  Demux3/2 -> Mux2/4
  [i_abc] -> Gain2/1
  [v_dq] -> PQ Calculation (dq-Frame)/1(vdq)  "v_dq"
  [i_dq_t] -> PQ Calculation (dq-Frame)/2(idq)  "i_dq"
  PQ Calculation (dq-Frame)/1(pq) -> [pq]
  [pq] -> Bus Creator/7  "pq"
  Gain1/1 -> [v_abc]
  Gain2/1 -> Demux1/1
  ia_m/1 -> Mux3/1
  ib_m/1 -> Mux3/2
  ic_m/1 -> Mux3/3
  Mux3/1 -> Gain3/1
  Gain3/1 -> [i_abc_t]
  [i_abc_t] -> "abc -> dq (Power-Invariant)1"/1(abc)
  [theta] -> "abc -> dq (Power-Invariant)1"/2(theta)
  "abc -> dq (Power-Invariant)1"/1(dq) -> [i_dq_t]
  Demux3/3 -> Mux2/5
  connections:
  vb/LConn2 -- va/LConn2 -- vc/LConn2 -- R_VD/RConn3 -- R_VD/RConn2 -- R_VD/RConn1 -- ia/RConn1 -- ib/RConn1 -- n/RConn1 -- ic/RConn1
  R_VD/LConn2 -- vb/LConn1 -- ib_m/RConn1 -- ib/LConn1
  R_VD/LConn3 -- ic/LConn1 -- ic_m/RConn1 -- vc/LConn1
  va/LConn1 -- R_VD/LConn1 -- ia/LConn1 -- ia_m/RConn1
  ia_m/LConn1 -- a/RConn1
  ib_m/LConn1 -- b/RConn1
  ic_m/LConn1 -- c/RConn1

== system SimplusGT/SynchronousMachineFull_Cyp_SMAVRPSSGOV (dq-Frame System Object) ==
  note: The actual current with considering discretization
  note: Synchronous machine IN Cyprus 14-bus system with AVR, PSS and GOV.
      |
      | Author(s): Yue Zhu
      |
      | Notes:
      |
      | This model is based on matlab system object.
      |
      | The model is in load convention.
      |
      | The frame transformation between dq and abc is done by simulink blocks, i.e., outside the system object.
  note: Matlab System Object
  note: Auxiliary
  note: Electrical Circuit
  Bus Creator : BusCreator  Inputs=7
  Constant2 : Constant  Value=OtherInputs
  Constant5 : Constant  Value=2*pi
  Demux : Demux
  Demux1 : Demux  Outputs=3
  Demux2 : Demux  Outputs=2
  Demux3 : Demux  Outputs=2
  Gain : Gain  Gain=1/Wbase
  Gain1 : Gain  Gain=1/Vbase
  Gain2 : Gain  Gain=Sbase/Vbase
  Gain3 : Gain  Gain=1/(Sbase/Vbase)
  MATLAB System : MATLABSystem  System=SimplusGT.Class.SynchronousMachineFull_Cyp_SMAVRPSSGOV  Ts=Ts  Para=ApparatusPara  ApparatusType=ApparatusType  PowerFlow=PowerFlow  x0=x0  DiscreMethod=DiscreMethod  LinearizationTimes=LinearizationTimes  DirectFeedthrough=DirectFeedthrough  VirtualResistor=DiscreDampingFlag  EquiInitial=true  ElecPortIOs=[ 1, 2 ]  SimulateUsing=Code generation
      mask Type: SimplusGT.Class.SynchronousMachineFull_Cyp_SMAVRPSSGOV
      mask Display:
      | disp('SynchronousMachineFull_Cyp_SMAVRPSSGOV');
      | port_label('input',1,'u');
      | port_label('output',1,'y');
  Math Function2 : Math  Operator=mod  SignedPower=on
  Mux : Mux  Inputs=2
  Mux1 : Mux  Inputs=3
  Mux2 : Mux
  Mux3 : Mux  Inputs=3
  PQ Calculation (dq-Frame) : Subsystem  AncestorBlock=|
      | SimplusGT/PQ Calculation
      | (dq-Frame)
      settings: LibrarySourceBlock=|
      | SimplusGT/PQ Calculation
      | (dq-Frame)
  R_VD : spsThreePhaseSeriesRLCBranchLib/Three-Phase Series RLC Branch  LConnTagsString=A|B|C  RConnTagsString=A|B|C  BranchType=R  Resistance=DiscreDampingValue*Vbase^2/Sbase  Inductance=1e-3  Capacitance=1e-6  Measurements=None
  "abc -> dq (Power-Invariant)" : Subsystem  AncestorBlock=|
      | SimplusGT/abc -> dq
      | (Power-Invariant)
      settings: LibrarySourceBlock=|
      | SimplusGT/abc -> dq
      | (Power-Invariant)
  "abc -> dq (Power-Invariant)1" : Subsystem  AncestorBlock=|
      | SimplusGT/abc -> dq
      | (Power-Invariant)
      settings: LibrarySourceBlock=|
      | SimplusGT/abc -> dq
      | (Power-Invariant)
  "dq -> abc (Power-Invariant)" : Subsystem  AncestorBlock=|
      | SimplusGT/dq -> abc
      | (Power-Invariant)
      settings: LibrarySourceBlock=|
      | SimplusGT/dq -> abc
      | (Power-Invariant)
  ia : spsControlledCurrentSourceLib/Controlled Current Source  Initialize=on  Source_Type=AC  Amplitude=0  Phase=0  Frequency=0  Measurements=None
  ia_m : spsCurrentMeasurementLib/Current Measurement  PhasorSimulation=off  OutputType=Complex  PSBequivalent=0
  ib : spsControlledCurrentSourceLib/Controlled Current Source  Initialize=on  Source_Type=AC  Amplitude=0  Phase=0  Frequency=0  Measurements=None
  ib_m : spsCurrentMeasurementLib/Current Measurement  PhasorSimulation=off  OutputType=Complex  PSBequivalent=0
  ic : spsControlledCurrentSourceLib/Controlled Current Source  Initialize=on  Source_Type=AC  Amplitude=0  Phase=0  Frequency=0  Measurements=None
  ic_m : spsCurrentMeasurementLib/Current Measurement  PhasorSimulation=off  OutputType=Complex  PSBequivalent=0
  va : spsVoltageMeasurementLib/Voltage Measurement  PhasorSimulation=off  OutputType=Complex  PSBequivalent=0
  vb : spsVoltageMeasurementLib/Voltage Measurement  PhasorSimulation=off  OutputType=Complex  PSBequivalent=0
  vc : spsVoltageMeasurementLib/Voltage Measurement  PhasorSimulation=off  OutputType=Complex  PSBequivalent=0
  a : PMIOPort  Side=Left
  b : PMIOPort  Port=2  Side=Left
  c : PMIOPort  Port=3  Side=Left
  n : PMIOPort  Port=4  Side=Left
  m : Outport
  wires:
  Demux/2 -> Mux/2
  Demux/1 -> Mux/1
  Mux/1 -> [i_dq]
  Demux/3 -> [w]
  Demux1/1 -> ia/1
  Demux1/2 -> ib/1
  va/1 -> Mux1/1
  vb/1 -> Mux1/2
  [v_dq] -> Demux2/1
  Demux2/1 -> Mux2/1
  Demux2/2 -> Mux2/2
  [v_abc] -> "abc -> dq (Power-Invariant)"/1(abc)
  [theta] -> "abc -> dq (Power-Invariant)"/2(theta)
  "abc -> dq (Power-Invariant)"/1(dq) -> [v_dq]
  [i_dq] -> "dq -> abc (Power-Invariant)"/1(dq)
  [theta] -> "dq -> abc (Power-Invariant)"/2(theta)
  "dq -> abc (Power-Invariant)"/1(abc) -> [i_abc]
  Mux2/1 -> MATLAB System/1
  MATLAB System/1 -> Demux/1
  vc/1 -> Mux1/3
  Demux1/3 -> ic/1
  Demux/4 -> Math Function2/1
  Constant5/1 -> Math Function2/2
  Math Function2/1 -> [theta]
  [v_dq] -> Bus Creator/1  "v_dq"
  [i_dq_t] -> Bus Creator/2  "i_dq"
  [v_abc] -> Bus Creator/3  "v_abc"
  [i_abc_t] -> Bus Creator/4  "i_abc"
  [w] -> Gain/1  "w"
  [theta] -> Bus Creator/6  "theta"
  Bus Creator/1 -> m/1
  Gain/1 -> Bus Creator/5  "w"
  Mux1/1 -> Gain1/1
  Constant2/1 -> Demux3/1
  Demux3/1 -> Mux2/3
  Demux3/2 -> Mux2/4
  [i_abc] -> Gain2/1
  [v_dq] -> PQ Calculation (dq-Frame)/1(vdq)  "v_dq"
  [i_dq_t] -> PQ Calculation (dq-Frame)/2(idq)  "i_dq"
  PQ Calculation (dq-Frame)/1(pq) -> [pq]
  [pq] -> Bus Creator/7  "pq"
  Gain1/1 -> [v_abc]
  Gain2/1 -> Demux1/1
  ia_m/1 -> Mux3/1
  ib_m/1 -> Mux3/2
  ic_m/1 -> Mux3/3
  Mux3/1 -> Gain3/1
  Gain3/1 -> [i_abc_t]
  [i_abc_t] -> "abc -> dq (Power-Invariant)1"/1(abc)
  [theta] -> "abc -> dq (Power-Invariant)1"/2(theta)
  "abc -> dq (Power-Invariant)1"/1(dq) -> [i_dq_t]
  connections:
  vb/LConn2 -- va/LConn2 -- vc/LConn2 -- R_VD/RConn3 -- R_VD/RConn2 -- R_VD/RConn1 -- ia/RConn1 -- ib/RConn1 -- n/RConn1 -- ic/RConn1
  R_VD/LConn2 -- vb/LConn1 -- ib_m/RConn1 -- ib/LConn1
  R_VD/LConn3 -- ic/LConn1 -- ic_m/RConn1 -- vc/LConn1
  va/LConn1 -- R_VD/LConn1 -- ia/LConn1 -- ia_m/RConn1
  ia_m/LConn1 -- a/RConn1
  ib_m/LConn1 -- b/RConn1
  ic_m/LConn1 -- c/RConn1

== system SimplusGT/SynchronousMachineFull_SM (dq-Frame System Object) ==
  note: The actual current with considering discretization
  note: Synchronous machine IN Cyprus 14-bus system with AVR, PSS and GOV.
      |
      | Author(s): Yue Zhu
      |
      | Notes:
      |
      | This model is based on matlab system object.
      |
      | The model is in load convention.
      |
      | The frame transformation between dq and abc is done by simulink blocks, i.e., outside the system object.
  note: Matlab System Object
  note: Auxiliary
  note: Electrical Circuit
  Bus Creator : BusCreator  Inputs=7
  Constant2 : Constant  Value=OtherInputs
  Constant5 : Constant  Value=2*pi
  Demux : Demux
  Demux1 : Demux  Outputs=3
  Demux2 : Demux  Outputs=2
  Demux3 : Demux  Outputs=2
  Gain : Gain  Gain=1/Wbase
  Gain1 : Gain  Gain=1/Vbase
  Gain2 : Gain  Gain=Sbase/Vbase
  Gain3 : Gain  Gain=1/(Sbase/Vbase)
  MATLAB System : MATLABSystem  System=SimplusGT.Class.SynchronousMachineFull_SM  Ts=Ts  Para=ApparatusPara  ApparatusType=ApparatusType  PowerFlow=PowerFlow  x0=x0  DiscreMethod=DiscreMethod  LinearizationTimes=LinearizationTimes  DirectFeedthrough=DirectFeedthrough  VirtualResistor=DiscreDampingFlag  EquiInitial=true  ElecPortIOs=[ 1, 2 ]  SimulateUsing=Code generation
      mask Type: SimplusGT.Class.SynchronousMachineFull_SM
      mask Display:
      | disp('SynchronousMachineFull_SM');
      | port_label('input',1,'u');
      | port_label('output',1,'y');
  Math Function2 : Math  Operator=mod  SignedPower=on
  Mux : Mux  Inputs=2
  Mux1 : Mux  Inputs=3
  Mux2 : Mux
  Mux3 : Mux  Inputs=3
  PQ Calculation (dq-Frame) : Subsystem  AncestorBlock=|
      | SimplusGT/PQ Calculation
      | (dq-Frame)
      settings: LibrarySourceBlock=|
      | SimplusGT/PQ Calculation
      | (dq-Frame)
  R_VD : spsThreePhaseSeriesRLCBranchLib/Three-Phase Series RLC Branch  LConnTagsString=A|B|C  RConnTagsString=A|B|C  BranchType=R  Resistance=DiscreDampingValue*Vbase^2/Sbase  Inductance=1e-3  Capacitance=1e-6  Measurements=None
  "abc -> dq (Power-Invariant)" : Subsystem  AncestorBlock=|
      | SimplusGT/abc -> dq
      | (Power-Invariant)
      settings: LibrarySourceBlock=|
      | SimplusGT/abc -> dq
      | (Power-Invariant)
  "abc -> dq (Power-Invariant)1" : Subsystem  AncestorBlock=|
      | SimplusGT/abc -> dq
      | (Power-Invariant)
      settings: LibrarySourceBlock=|
      | SimplusGT/abc -> dq
      | (Power-Invariant)
  "dq -> abc (Power-Invariant)" : Subsystem  AncestorBlock=|
      | SimplusGT/dq -> abc
      | (Power-Invariant)
      settings: LibrarySourceBlock=|
      | SimplusGT/dq -> abc
      | (Power-Invariant)
  ia : spsControlledCurrentSourceLib/Controlled Current Source  Initialize=on  Source_Type=AC  Amplitude=0  Phase=0  Frequency=0  Measurements=None
  ia_m : spsCurrentMeasurementLib/Current Measurement  PhasorSimulation=off  OutputType=Complex  PSBequivalent=0
  ib : spsControlledCurrentSourceLib/Controlled Current Source  Initialize=on  Source_Type=AC  Amplitude=0  Phase=0  Frequency=0  Measurements=None
  ib_m : spsCurrentMeasurementLib/Current Measurement  PhasorSimulation=off  OutputType=Complex  PSBequivalent=0
  ic : spsControlledCurrentSourceLib/Controlled Current Source  Initialize=on  Source_Type=AC  Amplitude=0  Phase=0  Frequency=0  Measurements=None
  ic_m : spsCurrentMeasurementLib/Current Measurement  PhasorSimulation=off  OutputType=Complex  PSBequivalent=0
  va : spsVoltageMeasurementLib/Voltage Measurement  PhasorSimulation=off  OutputType=Complex  PSBequivalent=0
  vb : spsVoltageMeasurementLib/Voltage Measurement  PhasorSimulation=off  OutputType=Complex  PSBequivalent=0
  vc : spsVoltageMeasurementLib/Voltage Measurement  PhasorSimulation=off  OutputType=Complex  PSBequivalent=0
  a : PMIOPort  Side=Left
  b : PMIOPort  Port=2  Side=Left
  c : PMIOPort  Port=3  Side=Left
  n : PMIOPort  Port=4  Side=Left
  m : Outport
  wires:
  Demux/2 -> Mux/2
  Demux/1 -> Mux/1
  Mux/1 -> [i_dq]
  Demux/3 -> [w]
  Demux1/1 -> ia/1
  Demux1/2 -> ib/1
  va/1 -> Mux1/1
  vb/1 -> Mux1/2
  [v_dq] -> Demux2/1
  Demux2/1 -> Mux2/1
  Demux2/2 -> Mux2/2
  [v_abc] -> "abc -> dq (Power-Invariant)"/1(abc)
  [theta] -> "abc -> dq (Power-Invariant)"/2(theta)
  "abc -> dq (Power-Invariant)"/1(dq) -> [v_dq]
  [i_dq] -> "dq -> abc (Power-Invariant)"/1(dq)
  [theta] -> "dq -> abc (Power-Invariant)"/2(theta)
  "dq -> abc (Power-Invariant)"/1(abc) -> [i_abc]
  Mux2/1 -> MATLAB System/1
  MATLAB System/1 -> Demux/1
  vc/1 -> Mux1/3
  Demux1/3 -> ic/1
  Demux/4 -> Math Function2/1
  Constant5/1 -> Math Function2/2
  Math Function2/1 -> [theta]
  [v_dq] -> Bus Creator/1  "v_dq"
  [i_dq_t] -> Bus Creator/2  "i_dq"
  [v_abc] -> Bus Creator/3  "v_abc"
  [i_abc_t] -> Bus Creator/4  "i_abc"
  [w] -> Gain/1  "w"
  [theta] -> Bus Creator/6  "theta"
  Bus Creator/1 -> m/1
  Gain/1 -> Bus Creator/5  "w"
  Mux1/1 -> Gain1/1
  Constant2/1 -> Demux3/1
  Demux3/1 -> Mux2/3
  Demux3/2 -> Mux2/4
  [i_abc] -> Gain2/1
  [v_dq] -> PQ Calculation (dq-Frame)/1(vdq)  "v_dq"
  [i_dq_t] -> PQ Calculation (dq-Frame)/2(idq)  "i_dq"
  PQ Calculation (dq-Frame)/1(pq) -> [pq]
  [pq] -> Bus Creator/7  "pq"
  Gain1/1 -> [v_abc]
  Gain2/1 -> Demux1/1
  ia_m/1 -> Mux3/1
  ib_m/1 -> Mux3/2
  ic_m/1 -> Mux3/3
  Mux3/1 -> Gain3/1
  Gain3/1 -> [i_abc_t]
  [i_abc_t] -> "abc -> dq (Power-Invariant)1"/1(abc)
  [theta] -> "abc -> dq (Power-Invariant)1"/2(theta)
  "abc -> dq (Power-Invariant)1"/1(dq) -> [i_dq_t]
  connections:
  vb/LConn2 -- va/LConn2 -- vc/LConn2 -- R_VD/RConn3 -- R_VD/RConn2 -- R_VD/RConn1 -- ia/RConn1 -- ib/RConn1 -- n/RConn1 -- ic/RConn1
  R_VD/LConn2 -- vb/LConn1 -- ib_m/RConn1 -- ib/LConn1
  R_VD/LConn3 -- ic/LConn1 -- ic_m/RConn1 -- vc/LConn1
  va/LConn1 -- R_VD/LConn1 -- ia/LConn1 -- ia_m/RConn1
  ia_m/LConn1 -- a/RConn1
  ib_m/LConn1 -- b/RConn1
  ic_m/LConn1 -- c/RConn1

== system SimplusGT/SynchronousMachineFull_SMAVR (dq-Frame System Object) ==
  note: The actual current with considering discretization
  note: Synchronous machine IN Cyprus 14-bus system with AVR, PSS and GOV.
      |
      | Author(s): Yue Zhu
      |
      | Notes:
      |
      | This model is based on matlab system object.
      |
      | The model is in load convention.
      |
      | The frame transformation between dq and abc is done by simulink blocks, i.e., outside the system object.
  note: Matlab System Object
  note: Auxiliary
  note: Electrical Circuit
  Bus Creator : BusCreator  Inputs=7
  Constant2 : Constant  Value=OtherInputs
  Constant5 : Constant  Value=2*pi
  Demux : Demux
  Demux1 : Demux  Outputs=3
  Demux2 : Demux  Outputs=2
  Demux3 : Demux  Outputs=2
  Gain : Gain  Gain=1/Wbase
  Gain1 : Gain  Gain=1/Vbase
  Gain2 : Gain  Gain=Sbase/Vbase
  Gain3 : Gain  Gain=1/(Sbase/Vbase)
  MATLAB System : MATLABSystem  System=SimplusGT.Class.SynchronousMachineFull_SMAVR  Ts=Ts  Para=ApparatusPara  ApparatusType=ApparatusType  PowerFlow=PowerFlow  x0=x0  DiscreMethod=DiscreMethod  LinearizationTimes=LinearizationTimes  DirectFeedthrough=DirectFeedthrough  VirtualResistor=DiscreDampingFlag  EquiInitial=true  ElecPortIOs=[ 1, 2 ]  SimulateUsing=Code generation
      mask Type: SimplusGT.Class.SynchronousMachineFull_SMAVR
      mask Display:
      | disp('SynchronousMachineFull_SMAVR');
      | port_label('input',1,'u');
      | port_label('output',1,'y');
  Math Function2 : Math  Operator=mod  SignedPower=on
  Mux : Mux  Inputs=2
  Mux1 : Mux  Inputs=3
  Mux2 : Mux
  Mux3 : Mux  Inputs=3
  PQ Calculation (dq-Frame) : Subsystem  AncestorBlock=|
      | SimplusGT/PQ Calculation
      | (dq-Frame)
      settings: LibrarySourceBlock=|
      | SimplusGT/PQ Calculation
      | (dq-Frame)
  R_VD : spsThreePhaseSeriesRLCBranchLib/Three-Phase Series RLC Branch  LConnTagsString=A|B|C  RConnTagsString=A|B|C  BranchType=R  Resistance=DiscreDampingValue*Vbase^2/Sbase  Inductance=1e-3  Capacitance=1e-6  Measurements=None
  "abc -> dq (Power-Invariant)" : Subsystem  AncestorBlock=|
      | SimplusGT/abc -> dq
      | (Power-Invariant)
      settings: LibrarySourceBlock=|
      | SimplusGT/abc -> dq
      | (Power-Invariant)
  "abc -> dq (Power-Invariant)1" : Subsystem  AncestorBlock=|
      | SimplusGT/abc -> dq
      | (Power-Invariant)
      settings: LibrarySourceBlock=|
      | SimplusGT/abc -> dq
      | (Power-Invariant)
  "dq -> abc (Power-Invariant)" : Subsystem  AncestorBlock=|
      | SimplusGT/dq -> abc
      | (Power-Invariant)
      settings: LibrarySourceBlock=|
      | SimplusGT/dq -> abc
      | (Power-Invariant)
  ia : spsControlledCurrentSourceLib/Controlled Current Source  Initialize=on  Source_Type=AC  Amplitude=0  Phase=0  Frequency=0  Measurements=None
  ia_m : spsCurrentMeasurementLib/Current Measurement  PhasorSimulation=off  OutputType=Complex  PSBequivalent=0
  ib : spsControlledCurrentSourceLib/Controlled Current Source  Initialize=on  Source_Type=AC  Amplitude=0  Phase=0  Frequency=0  Measurements=None
  ib_m : spsCurrentMeasurementLib/Current Measurement  PhasorSimulation=off  OutputType=Complex  PSBequivalent=0
  ic : spsControlledCurrentSourceLib/Controlled Current Source  Initialize=on  Source_Type=AC  Amplitude=0  Phase=0  Frequency=0  Measurements=None
  ic_m : spsCurrentMeasurementLib/Current Measurement  PhasorSimulation=off  OutputType=Complex  PSBequivalent=0
  va : spsVoltageMeasurementLib/Voltage Measurement  PhasorSimulation=off  OutputType=Complex  PSBequivalent=0
  vb : spsVoltageMeasurementLib/Voltage Measurement  PhasorSimulation=off  OutputType=Complex  PSBequivalent=0
  vc : spsVoltageMeasurementLib/Voltage Measurement  PhasorSimulation=off  OutputType=Complex  PSBequivalent=0
  a : PMIOPort  Side=Left
  b : PMIOPort  Port=2  Side=Left
  c : PMIOPort  Port=3  Side=Left
  n : PMIOPort  Port=4  Side=Left
  m : Outport
  wires:
  Demux/2 -> Mux/2
  Demux/1 -> Mux/1
  Mux/1 -> [i_dq]
  Demux/3 -> [w]
  Demux1/1 -> ia/1
  Demux1/2 -> ib/1
  va/1 -> Mux1/1
  vb/1 -> Mux1/2
  [v_dq] -> Demux2/1
  Demux2/1 -> Mux2/1
  Demux2/2 -> Mux2/2
  [v_abc] -> "abc -> dq (Power-Invariant)"/1(abc)
  [theta] -> "abc -> dq (Power-Invariant)"/2(theta)
  "abc -> dq (Power-Invariant)"/1(dq) -> [v_dq]
  [i_dq] -> "dq -> abc (Power-Invariant)"/1(dq)
  [theta] -> "dq -> abc (Power-Invariant)"/2(theta)
  "dq -> abc (Power-Invariant)"/1(abc) -> [i_abc]
  Mux2/1 -> MATLAB System/1
  MATLAB System/1 -> Demux/1
  vc/1 -> Mux1/3
  Demux1/3 -> ic/1
  Demux/4 -> Math Function2/1
  Constant5/1 -> Math Function2/2
  Math Function2/1 -> [theta]
  [v_dq] -> Bus Creator/1  "v_dq"
  [i_dq_t] -> Bus Creator/2  "i_dq"
  [v_abc] -> Bus Creator/3  "v_abc"
  [i_abc_t] -> Bus Creator/4  "i_abc"
  [w] -> Gain/1  "w"
  [theta] -> Bus Creator/6  "theta"
  Bus Creator/1 -> m/1
  Gain/1 -> Bus Creator/5  "w"
  Mux1/1 -> Gain1/1
  Constant2/1 -> Demux3/1
  Demux3/1 -> Mux2/3
  Demux3/2 -> Mux2/4
  [i_abc] -> Gain2/1
  [v_dq] -> PQ Calculation (dq-Frame)/1(vdq)  "v_dq"
  [i_dq_t] -> PQ Calculation (dq-Frame)/2(idq)  "i_dq"
  PQ Calculation (dq-Frame)/1(pq) -> [pq]
  [pq] -> Bus Creator/7  "pq"
  Gain1/1 -> [v_abc]
  Gain2/1 -> Demux1/1
  ia_m/1 -> Mux3/1
  ib_m/1 -> Mux3/2
  ic_m/1 -> Mux3/3
  Mux3/1 -> Gain3/1
  Gain3/1 -> [i_abc_t]
  [i_abc_t] -> "abc -> dq (Power-Invariant)1"/1(abc)
  [theta] -> "abc -> dq (Power-Invariant)1"/2(theta)
  "abc -> dq (Power-Invariant)1"/1(dq) -> [i_dq_t]
  connections:
  vb/LConn2 -- va/LConn2 -- vc/LConn2 -- R_VD/RConn3 -- R_VD/RConn2 -- R_VD/RConn1 -- ia/RConn1 -- ib/RConn1 -- n/RConn1 -- ic/RConn1
  R_VD/LConn2 -- vb/LConn1 -- ib_m/RConn1 -- ib/LConn1
  R_VD/LConn3 -- ic/LConn1 -- ic_m/RConn1 -- vc/LConn1
  va/LConn1 -- R_VD/LConn1 -- ia/LConn1 -- ia_m/RConn1
  ia_m/LConn1 -- a/RConn1
  ib_m/LConn1 -- b/RConn1
  ic_m/LConn1 -- c/RConn1
